simulink model "Q4"  (R2020b)
settings: Solver=VariableStepAuto  StartTime=0.0  StopTime=30  RelTol=1e-3
undefined symbols (not defined in the file): A_num, B_num, C_num, k1_integ, k2_integ
libraries: simulink x1
settings Model: Creator=asus  LastModifiedBy=asus

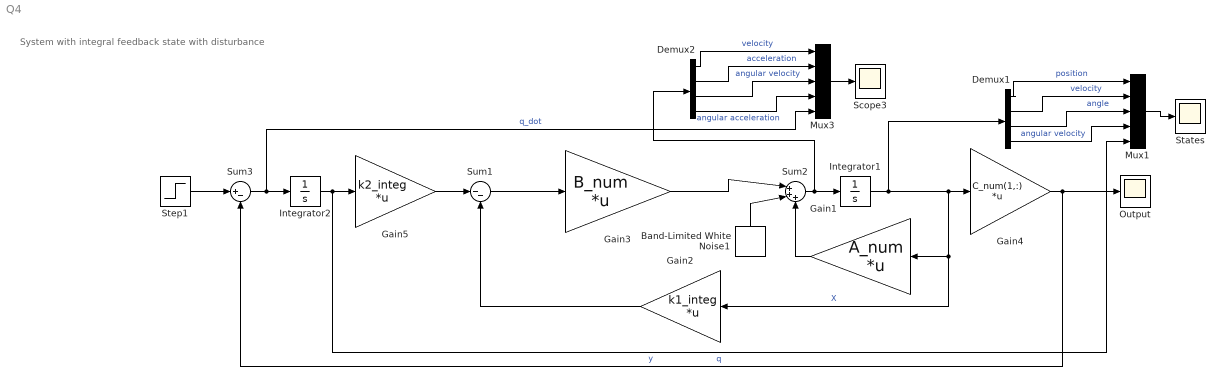
== system Q4 ==
  note: System with integral feedback state with disturbance
  Band-Limited White Noise1 : simulink/Sources/Band-Limited White Noise  Cov=[0.3; 0.3; 0.3; 0.3]  Ts=20  seed=[456; 456; 456; 456]
  Demux1 : Demux
  Demux2 : Demux
  Gain1 : Gain  Gain=A_num  Multiplication=Matrix(K*u)
  Gain2 : Gain  Gain=k1_integ  Multiplication=Matrix(K*u)
  Gain3 : Gain  Gain=B_num  Multiplication=Matrix(K*u)
  Gain4 : Gain  Gain=C_num(1,:)  Multiplication=Matrix(K*u)
  Gain5 : Gain  Gain=k2_integ  Multiplication=Matrix(K*u)
  Integrator1 : Integrator
  Integrator2 : Integrator
  Mux1 : Mux  Inputs=5
  Mux3 : Mux  Inputs=5
  Output : Scope
  Scope3 : Scope
  States : Scope
  Step1 : Step  After=0.1  SampleTime=0
  Sum1 : Sum  Inputs=|--
  Sum2 : Sum  Inputs=|+++
  Sum3 : Sum  Inputs=|+-
  wires:
  Gain5/1 -> Sum1/1
  Gain2/1 -> Sum1/2
  Mux3/1 -> Scope3/1
  Sum2/1 -> Demux2/1, Integrator1/1
  Demux2/4 -> Mux3/4  "angular acceleration"
  Gain4/1 -> Sum3/2, Output/1  "y"
  Mux1/1 -> States/1
  Demux2/1 -> Mux3/1  "velocity"
  Demux1/4 -> Mux1/4  "angular velocity"
  Integrator2/1 -> Mux1/5, Gain5/1  "q"
  Sum3/1 -> Mux3/5, Integrator2/1  "q_dot"
  Integrator1/1 -> Gain2/1, Gain1/1, Gain4/1, Demux1/1  "X"
  Demux1/1 -> Mux1/1  "position"
  Demux1/2 -> Mux1/2  "velocity"
  Gain3/1 -> Sum2/1
  Demux2/2 -> Mux3/2  "acceleration"
  Step1/1 -> Sum3/1
  Demux1/3 -> Mux1/3  "angle"
  Demux2/3 -> Mux3/3  "angular velocity"
  Sum1/1 -> Gain3/1
  Gain1/1 -> Sum2/3
  Band-Limited White Noise1/1 -> Sum2/2
